simulink model ""  (R2025b)
settings: Solver=VariableStepAuto  StartTime=0.0  StopTime=20  RelTol=1e-3
undefined symbols (not defined in the file): k1, k2, k3, k4, limite_inf_att, limite_sup_att, tau_derivatore
settings Model: Creator=USER  LastModifiedBy=francesco
settings SolverCC: AlgebraicLoopSolver=TrustRegion
settings DebuggingCC: AlgebraicLoopMsg=none  UnconnectedInputMsg=warning  UnconnectedOutputMsg=warning  UnconnectedLineMsg=warning
settings ModelReferenceCC: EnableRefExpFcnMdlSchedulingChecks=on
settings RTWCC: GPUComputeCapability=3.5  DLArmComputeVersion=19.05

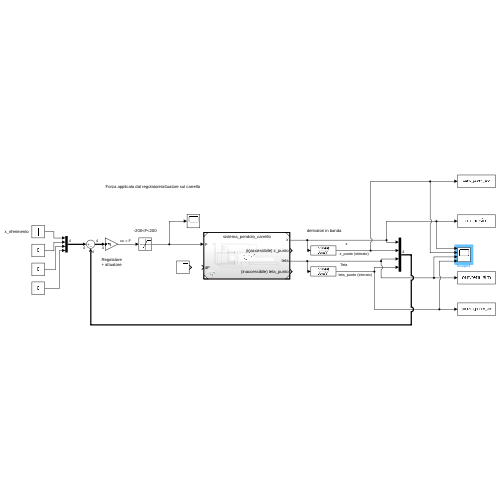
[thumbnail: Simulink's stored preview of the top-level diagram]
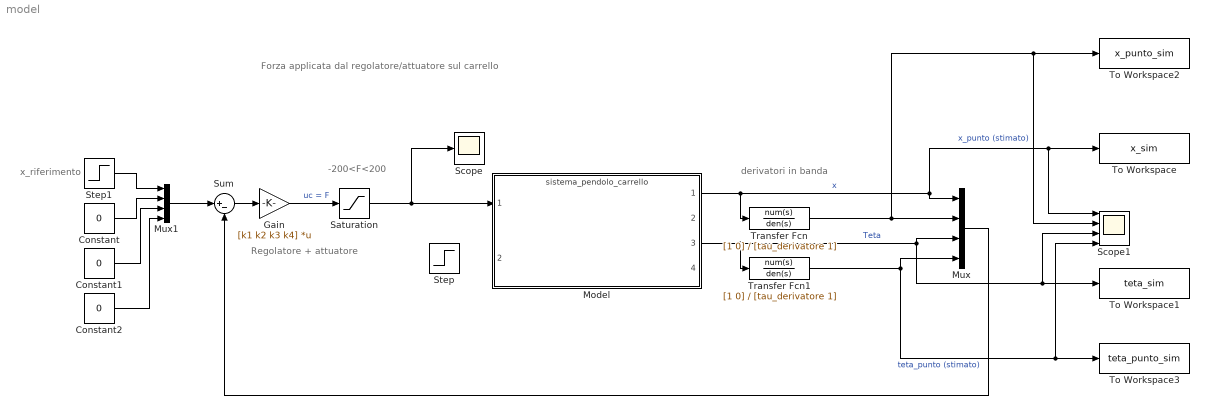
== system model ==
  note: x_riferimento
  note: derivatori in banda
  note: -200<F<200
  note: Regolatore
      | + attuatore
  note: Forza applicata dal regolatore/attuatore sul carrello
  Constant : Constant  Value=0
  Constant1 : Constant  Value=0
  Constant2 : Constant  Value=0
  Gain : Gain  Gain=[k1 k2 k3 k4]  Multiplication=Matrix(K*u)
  Model : ModelReference  ModelNameDialog=sistema_pendolo_carrello.slx  SimulationMode=Normal  ModelReferenceVersion=9.29
  Mux : Mux
  Mux1 : Mux
  Saturation : Saturate  UpperLimit=limite_sup_att  LowerLimit=limite_inf_att
  Scope : Scope
  Scope1 : Scope  NumInputPorts=4
      settings: ActiveDisplayString=4  ActiveDisplayYMinimum=-0.39414045873539633  ActiveDisplayYMaximum=0.17993077782329631
  Step : Step  SampleTime=0
  Step1 : Step  After=5  SampleTime=0
  Sum : Sum  Inputs=|+-
  To Workspace : ToWorkspace  VariableName=x_sim  SaveFormat=Timeseries  SampleTime=-1
  To Workspace1 : ToWorkspace  VariableName=teta_sim  SaveFormat=Timeseries  SampleTime=-1
  To Workspace2 : ToWorkspace  VariableName=x_punto_sim  SaveFormat=Timeseries  SampleTime=-1
  To Workspace3 : ToWorkspace  VariableName=teta_punto_sim  SaveFormat=Timeseries  SampleTime=-1
  Transfer Fcn : TransferFcn  Numerator=[1 0]  Denominator=[tau_derivatore 1]
  Transfer Fcn1 : TransferFcn  Numerator=[1 0]  Denominator=[tau_derivatore 1]
  wires:
  Gain/1 -> Saturation/1  "uc = F"
  Model/1 -> Mux/1, Scope1/1, To Workspace/1, Transfer Fcn/1  "x"
  Model/3 -> Transfer Fcn1/1, Scope1/3, To Workspace1/1, Mux/3  "Teta"
  Saturation/1 -> Model/1, Scope/1
  Transfer Fcn/1 -> Mux/2, To Workspace2/1, Scope1/2  "x_punto (stimato)"
  Transfer Fcn1/1 -> Mux/4, Scope1/4, To Workspace3/1  "teta_punto (stimato)"
  Sum/1 -> Gain/1
  Mux/1 -> Sum/2
  Step1/1 -> Mux1/1
  Constant/1 -> Mux1/2
  Constant1/1 -> Mux1/3
  Constant2/1 -> Mux1/4
  Mux1/1 -> Sum/1
